simulink model "TestSoundWAV"  (Simulink 6.4)
settings: Solver=FixedStepDiscrete  SolverMode=SingleTasking  StartTime=0  StopTime=inf  FixedStep=0.001  RelTol=1e-3
PreLoadFcn:
  | FrequencyList
libraries: ecrobot_nxt_lib x5
CloseFcn:
  | rtwprivate ssgencode ModelCloseRequest TestBluetooth
settings Model: Creator=tchikama  LastModifiedBy=tchikama  ProdHWDeviceType=ARM7
settings DataIOCC: SaveOutput=off  SignalLogging=off  SaveTime=off
settings OptimizationCC: InlineParams=on  InlineInvariantSignals=on  RollThreshold=2  StateBitsets=on  DataBitsets=on  UseTempVars=on  InitFltsAndDblsToZero=off  NoFixptDivByZeroProtection=on  EfficientFloat2IntCast=on  OptimizeModelRefInitCode=on  LifeSpan=1
settings DebuggingCC: ConsistencyChecking=warning  SignalInfNanChecking=warning  ReadBeforeWriteMsg=DisableAll  WriteAfterWriteMsg=DisableAll  WriteAfterReadMsg=DisableAll  AlgebraicLoopMsg=error  CheckExecutionContextPreStartOutputMsg=on  CheckExecutionContextRuntimeOutputMsg=on  SolverPrmCheckMsg=none  SingleTaskRateTransMsg=warning  TasksWithSamePriorityMsg=none  IntegerOverflowMsg=error  ParameterPrecisionLossMsg=none  UnconnectedInputMsg=error  UnconnectedOutputMsg=error  UnconnectedLineMsg=error  UniqueDataStoreMsg=error  BusObjectLabelMismatch=error  RootOutportRequireBusObject=error  ModelReferenceIOMsg=warning  ModelReferenceVersionMismatchMessage=warning  ModelReferenceIOMismatchMessage=warning
settings HardwareCC: ProdIntDivRoundTo=Zero  ProdEndianess=LittleEndian  ProdHWDeviceType=ARM7  TargetHWDeviceType=32-bit Generic
settings ModelReferenceCC: ModelReferenceNumInstancesAllowed=Single
settings RTWCC: SystemTargetFile=ert.tlc  GenCodeOnly=on  GenerateMakefile=off  TemplateMakefile=ert_default_tmf  Description=Real-Time Workshop Embedded Coder (no auto configuration)  GenerateReport=on  RTWVerbose=off  ProcessScript=ert_make_rtw_hook  IncludeHyperlinkInReport=on  LaunchReport=on
settings CodeAppCC: ForceParamTrailComments=on  IgnoreCustomStorageClasses=off  SFDataObjDesc=on  PrefixModelToSubsysFcnNames=off  CustomSymbolStrGlobalVar=rt$N$M  CustomSymbolStrType=$N$M  CustomSymbolStrFcn=$N$M$F  CustomSymbolStrMacro=$N$M  InsertBlockDesc=on
settings ERTTargetCC: TargetFcnLib=ansi_tfl_tmw.mat  GenFloatMathFcnCalls=GNU  IncludeMdlTerminateFcn=off  SuppressErrorStatus=on  IncludeERTFirstTime=on  SupportAbsoluteTime=off  SupportNonFinite=off  SupportComplex=off  PurelyIntegerCode=on  InlinedParameterPlacement=NonHierarchical  RootIOFormat=Structure reference  ERTCustomFileTemplate=example_file_process.tlc  InitialValueSource=Model

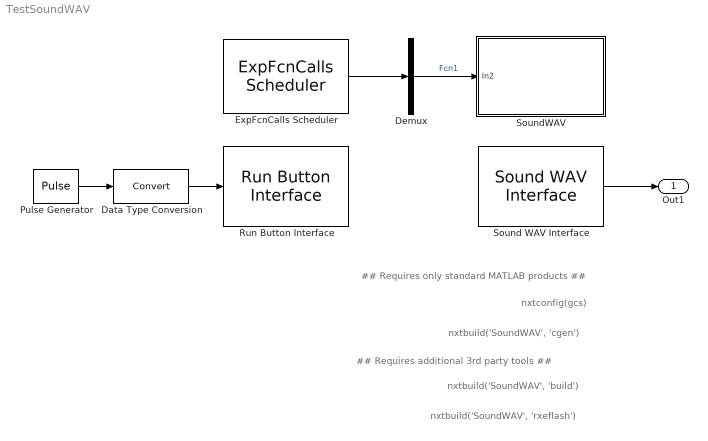
== system TestSoundWAV ==
  note: nxtbuild('SoundWAV', 'build')
  note: nxtbuild('SoundWAV', 'rxeflash')
  note: nxtbuild('SoundWAV', 'cgen')
  note: ## Requires only standard MATLAB products ##
  note: ## Requires additional 3rd party tools ##
  note: nxtconfig(gcs)
  Data Type Conversion : DataTypeConversion
  Demux : Demux  Outputs=1
  ExpFcnCalls Scheduler : ecrobot_nxt_lib/ExpFcnCalls Scheduler  Priority=1  fcname='Fcn1'  fctrigger=[10]  ts=0.001  platform=OSEK  stacksize=[512]  bd_mode=Slave  bd_addr='00', '16', '53', '04', 'F1', 'B3', '00'
  Pulse Generator : DiscretePulseGenerator  Period=100  PulseWidth=50  SampleTime=0.001
  Run Button Interface : ecrobot_nxt_lib/Run Button Interface  SystemSampleTime=-1
  Sound WAV Interface : ecrobot_nxt_lib/Sound WAV Interface  SystemSampleTime=-1  wav='mtlb'
  SoundWAV : Subsystem
  Out1 : Outport
  wires:
  ExpFcnCalls Scheduler/1 -> Demux/1
  Sound WAV Interface/1 -> Out1/1
  Pulse Generator/1 -> Data Type Conversion/1
  Demux/1 -> SoundWAV/1(In2)  "Fcn1"
  Data Type Conversion/1 -> Run Button Interface/1

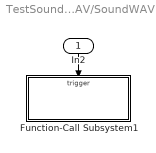
== system TestSoundWAV/SoundWAV ==
  In2 : Inport  Orientation=down
  Function-Call Subsystem1 : Subsystem  TreatAsAtomicUnit=on
  wires:
  In2/1 -> Function-Call Subsystem1/Trigger

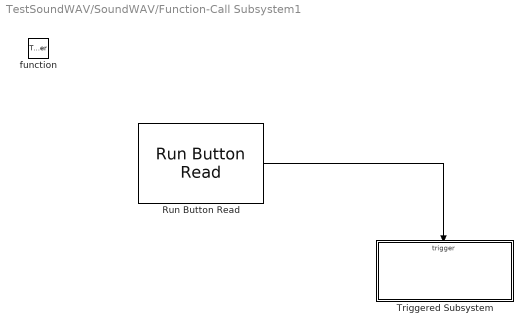
== system TestSoundWAV/SoundWAV/Function-Call Subsystem1 ==
  function : TriggerPort  TriggerType=function-call
  Run Button Read : ecrobot_nxt_lib/Run Button Read  SystemSampleTime=-1
  Triggered Subsystem : Subsystem  TreatAsAtomicUnit=on
  wires:
  Run Button Read/1 -> Triggered Subsystem/Trigger

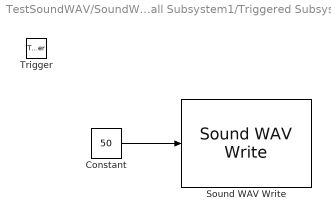
== system TestSoundWAV/SoundWAV/Function-Call Subsystem1/Triggered Subsystem ==
  Trigger : TriggerPort
  Constant : Constant  Value=50  OutDataType=sfix(16)  ConRadixGroup=Use specified scaling  OutScaling=2^0  SampleTime=inf  FramePeriod=inf
  Sound WAV Write : ecrobot_nxt_lib/Sound WAV Write  SystemSampleTime=-1  wav='mtlb'
  wires:
  Constant/1 -> Sound WAV Write/1
